simulink model "lowpassfilt"  (R2017a)
settings: Solver=VariableStepAuto  StartTime=0.0  StopTime=.5  RelTol=1e-3
libraries: fl_lib x5, nesl_utility x3
settings Model: Creator=b  LastModifiedBy=b

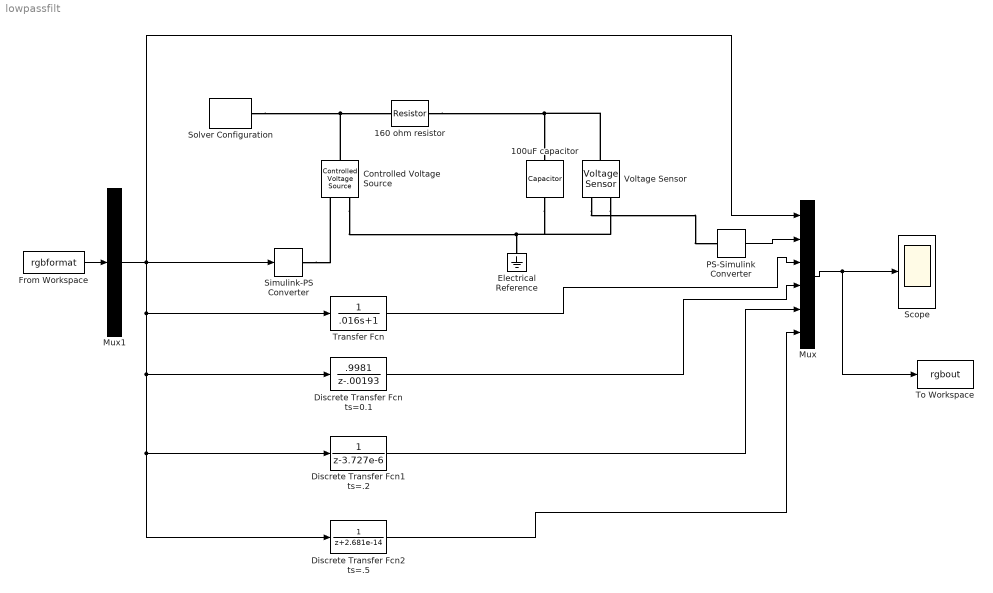
== system lowpassfilt ==
  "100uF capacitor " : fl_lib/Electrical/Electrical Elements/Capacitor  c=100 uF  r=1e-6 Ohm  g=0 1/Ohm  i_specify=off  i_priority=None  i=0 A  i_nominal_specify=off  i_nominal_unit=A  i_nominal_value=1  v_specify=off  v_priority=None  v=0 V  v_nominal_specify=off  v_nominal_unit=V  v_nominal_value=1  vc_specify=off  vc_priority=High  vc=0 V  vc_nominal_specify=off  vc_nominal_unit=V  vc_nominal_value=1
  160 ohm resistor : fl_lib/Electrical/Electrical Elements/Resistor  R=160 Ohm  i_specify=off  i_priority=None  i=0 A  i_nominal_specify=off  i_nominal_unit=A  i_nominal_value=1  v_specify=off  v_priority=None  v=0 V  v_nominal_specify=off  v_nominal_unit=V  v_nominal_value=1
  Controlled Voltage Source : fl_lib/Electrical/Electrical Sources/Controlled Voltage Source
  "Discrete Transfer Fcn ts=0.1 " : DiscreteTransferFcn  Numerator=[.9981]  Denominator=[1 -.00193]
  "Discrete Transfer Fcn1 ts=.2 " : DiscreteTransferFcn  Denominator=[1 -3.727e-6]
  Discrete Transfer Fcn2 ts=.5 : DiscreteTransferFcn  Denominator=[1 2.681e-14]
  Electrical Reference : fl_lib/Electrical/Electrical Elements/Electrical Reference
  From Workspace : FromWorkspace  VariableName=rgbformat  SampleTime=0
  Mux : Mux  Inputs=6
  Mux1 : Mux  Inputs=1
  PS-Simulink Converter : nesl_utility/PS-Simulink Converter  PhysicalDomain=network_engine_domain  SubClassName=ps_output  LeftPortType=input  RightPortType=output  PseudoPeriodic=off  Frequencies=[]  Unit=1  AffineConversion=off
  Scope : Scope
  Simulink-PS Converter : nesl_utility/Simulink-PS Converter  PhysicalDomain=network_engine_domain  SubClassName=ps_input  LeftPortType=input  RightPortType=output  PseudoPeriodic=off  Frequencies=[]  NoiseDistribution=none  NoiseParameters=[]  Unit=1  AffineConversion=off  FilteringAndDerivatives=provide  SimscapeFilterOrder=1  InputFilterTimeConstant=0.001  UdotUserProvided=0
  Solver Configuration : nesl_utility/Solver Configuration  PhysicalDomain=network_engine_domain  SubClassName=solver  LeftPortType=input  RightPortType=generic  Accelerate=off  Tones=[]  Harmonics=[]  SimulateNoise=off  Profile=off  UseLocalSampling=off  EnableSwitchedLinearOptims=on  FrequencyDomain=off  UseCCode=off  RelTol=0.001  AbsTol=1e-06  MinStep=1e-09  ToWorkspace=off  RevertToSquareIcSolve=off  NumHomotopyIterations=100  PhasorMode=off  PhasorModeNumHarmonics=1  OverrideAbsTol=off  DoDC=off  ResidualTolerance=.01  UseLocalSolver=off  LocalSolverChoice=NE_BACKWARD_EULER_ADVANCER  LocalSolverSampleTime=0.001  DoFixedCost=off  MaxNonlinIter=3  MaxModeIter=2  LinearAlgebra=Sparse  DelaysMemoryBudget=1024  AutomaticFiltering=on  FilteringTimeConstant=0.001
  To Workspace : ToWorkspace  VariableName=rgbout  SaveFormat=Timeseries  SampleTime=-1
  Transfer Fcn : TransferFcn  Denominator=[.016 1]
  Voltage Sensor : fl_lib/Electrical/Electrical Sensors/Voltage Sensor
  wires:
  PS-Simulink Converter/1 -> Mux/2
  From Workspace/1 -> Mux1/1
  Mux1/1 -> Mux/1, Discrete Transfer Fcn2 ts=.5/1, "Discrete Transfer Fcn1 ts=.2 "/1, "Discrete Transfer Fcn ts=0.1 "/1, Transfer Fcn/1, Simulink-PS Converter/1
  Transfer Fcn/1 -> Mux/3
  "Discrete Transfer Fcn ts=0.1 "/1 -> Mux/4
  "Discrete Transfer Fcn1 ts=.2 "/1 -> Mux/5
  Mux/1 -> To Workspace/1, Scope/1
  Discrete Transfer Fcn2 ts=.5/1 -> Mux/6
  connections:
  160 ohm resistor/RConn1 -- Voltage Sensor/LConn1 -- "100uF capacitor "/LConn1
  Simulink-PS Converter/RConn1 -- Controlled Voltage Source/RConn1
  Controlled Voltage Source/LConn1 -- 160 ohm resistor/LConn1 -- Solver Configuration/RConn1
  Controlled Voltage Source/RConn2 -- Voltage Sensor/RConn2 -- "100uF capacitor "/RConn1 -- Electrical Reference/LConn1
  Voltage Sensor/RConn1 -- PS-Simulink Converter/LConn1
